simulink model "gm_opv_pluto_transmitter_HDL_coder_input"  (R2023a)
settings: Solver=FixedStepDiscrete  StartTime=0.0  StopTime=.02*40e-3  RelTol=1e-3
undefined symbols (not defined in the file or in its folder): bit_rate, bits_per_symbol, device_clock, PTTlength, symbol_rate
libraries: dsphdlsigops2 x2, hdlsllib x2, dspindex x1, commrandsrc3 x1
settings Model: Creator=matt  LastModifiedBy=matt
settings OptimizationCC: BlockReduction=off  ConditionallyExecuteInputs=off  DefaultParameterBehavior=Inlined
settings DebuggingCC: AlgebraicLoopMsg=error  InheritedTsInSrcMsg=none
settings HardwareCC: ProdBitPerPointer=32  ProdBitPerSizeT=32  ProdBitPerPtrDiffT=32  ProdLargestAtomicFloat=None  ProdIntDivRoundTo=Undefined  ProdEndianess=Unspecified  ProdWordSize=32  ProdHWDeviceType=ASIC/FPGA->ASIC/FPGA  TargetBitPerLong=64  TargetBitPerPointer=64  TargetBitPerSizeT=64  TargetBitPerPtrDiffT=64  TargetLongLongMode=on  TargetIntDivRoundTo=Zero  TargetEndianess=LittleEndian  TargetWordSize=64  TargetHWDeviceType=Custom Processor->MATLAB Host Computer  ProdEqTarget=off

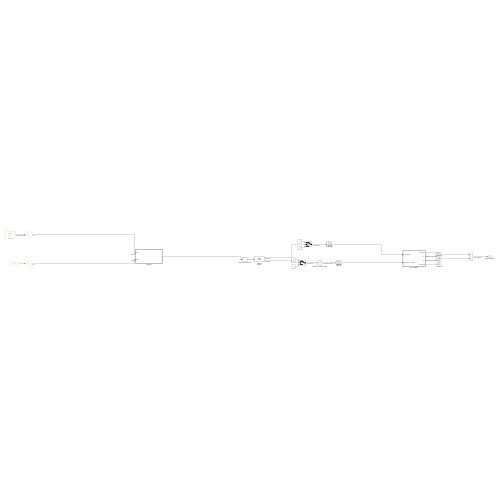
[thumbnail: Simulink's stored preview of the top-level diagram]
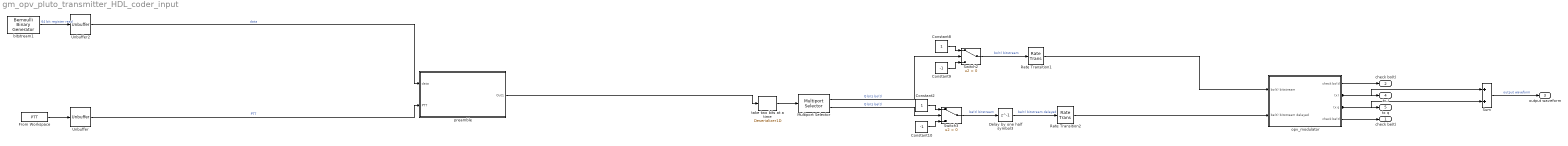
== system gm_opv_pluto_transmitter_HDL_coder_input ==
  Constant10 : Constant  Value=-1  OutDataTypeStr=fixdt(1,16,15)
  Constant2 : Constant  OutDataTypeStr=fixdt(1,16,15)
  Constant8 : Constant  OutDataTypeStr=fixdt(1,16,15)
  Constant9 : Constant  Value=-1  OutDataTypeStr=fixdt(1,16,15)
  Delay by one half symbol3 : Delay  DelayLength=1  SampleTime=1/(bits_per_symbol*symbol_rate)
  From Workspace : FromWorkspace  VariableName=PTT  SampleTime=PTTlength/(bit_rate)
  Multiport Selector : dspindex/Multiport Selector  rowsOrCols=Rows  idxCellArray={ 1, 2 }  idxErrMode=Clip Index
      settings: LibrarySourceBlock=|
      | dsphdlsupportsigmgmt/Multiport
      | Selector
  Rate Transition1 : RateTransition  Deterministic=off  OutPortSampleTime=1/device_clock
  Rate Transition2 : RateTransition  Deterministic=off  OutPortSampleTime=1/device_clock
  Sum : Sum  OutDataTypeStr=fixdt(1,16,15)  SaturateOnIntegerOverflow=on
  Switch2 : Switch  Criteria=u2 > Threshold  OutDataTypeStr=fixdt(1,16,15)  SaturateOnIntegerOverflow=off  InputSameDT=off
  Switch3 : Switch  Criteria=u2 > Threshold  OutDataTypeStr=fixdt(1,16,15)  SaturateOnIntegerOverflow=off  InputSameDT=off
  Unbuffer : Unbuffer
  Unbuffer2 : Unbuffer
  bitstream1 : commrandsrc3/Bernoulli Binary Generator  ProbabilityOfZero=0.5  SeedSource=Auto  Seed=0  SampleTime=(1/bit_rate)  SamplesPerFrame=64  OutputDataType=boolean  SimulateUsing=Interpreted execution
  opv_modulator : Subsystem  TreatAsAtomicUnit=on
  preamble : Subsystem  TreatAsAtomicUnit=on
  take two bits at a time : hdlsllib/HDL Operations/Deserializer1D  Ratio=2  IdleCycles=0  InitialCondition=0  startIn=off  validIn=off  validOut=off  inputDataDimensions=-1  inputSampleTime=-1  inputSignalType=auto
  check be(t) : Outport
  "check bo(t) " : Outport  Port=2
  output waveform : Outport  Port=3
  tx I : Outport  Port=4
  tx q : Outport  Port=5
  wires:
  preamble/1(Out1) -> take two bits at a time/1
  Unbuffer/1 -> preamble/2(PTT)  "PTT"
  Unbuffer2/1 -> preamble/1(data)  "data"
  opv_modulator/4(check be(t)) -> check be(t)/1
  opv_modulator/3(tx q) -> tx q/1, Sum/2
  opv_modulator/2(tx I) -> tx I/1, Sum/1
  opv_modulator/1("check bo(t) ") -> "check bo(t) "/1
  Rate Transition2/1 -> opv_modulator/2(be(t) bitstream delayed)
  Rate Transition1/1 -> opv_modulator/1(bo(t) bitstream)
  bitstream1/1 -> Unbuffer2/1  "64 bit register read"
  Constant2/1 -> Switch3/1
  Constant10/1 -> Switch3/3
  Constant9/1 -> Switch2/3
  Constant8/1 -> Switch2/1
  Multiport Selector/2 -> Switch3/2  "Q bits be(t)"
  Multiport Selector/1 -> Switch2/2  "Q bits bo(t)"
  take two bits at a time/1 -> Multiport Selector/1
  From Workspace/1 -> Unbuffer/1
  Delay by one half symbol3/1 -> Rate Transition2/1  "be(t) bitstream delayed"
  Sum/1 -> output waveform/1  "output waveform"
  Switch3/1 -> Delay by one half symbol3/1  "be(t) bitstream"
  Switch2/1 -> Rate Transition1/1  "bo(t) bitstream"

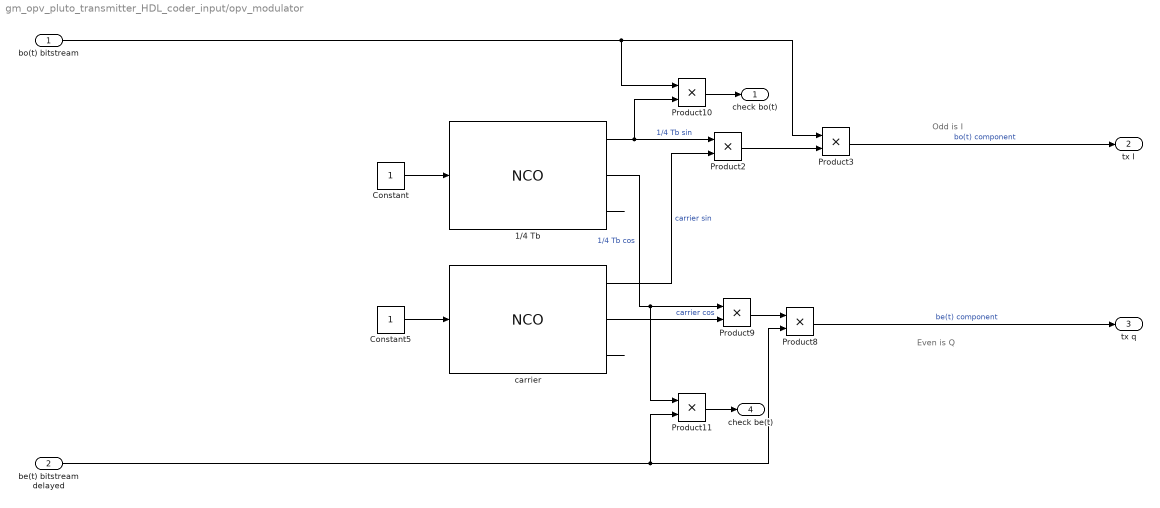
== system gm_opv_pluto_transmitter_HDL_coder_input/opv_modulator ==
  note: Odd is I
  note: Even is Q
  bo(t) bitstream : Inport
  be(t) bitstream delayed : Inport  Port=2
  1/4 Tb : dsphdlsigops2/NCO  PhaseIncrementSource=Property  PhaseIncrement=phase_increment_bo_be  PhaseOffsetSource=Property  PhaseOffset=phase_offset  DitherSource=None  NumDitherBits=dither_bits  SamplesPerFrame=1  LUTCompress=on  ResetAction=off  Waveform=Sine and cosine  PhasePort=off  SimulateUsing=Code generation  AccumulatorWL=accumulator_width  PhaseQuantization=on  NumQuantizerAccumulatorBits=quantizer_word_length  OutputDataType=Binary point scaling  OutputWL=16  OutputFL=15
      settings: LibrarySourceBlock=dsphdlsrcs2/NCO
  Constant : Constant  OutDataTypeStr=boolean
  Constant5 : Constant  OutDataTypeStr=boolean
  Product{2..3,8..11} (6 alike) : Product  OutDataTypeStr=fixdt(1,16,15)
  carrier : dsphdlsigops2/NCO  PhaseIncrementSource=Property  PhaseIncrement=phase_increment_carrier  PhaseOffsetSource=Property  PhaseOffset=phase_offset  DitherSource=None  NumDitherBits=dither_bits  SamplesPerFrame=1  LUTCompress=on  ResetAction=off  Waveform=Sine and cosine  PhasePort=off  SimulateUsing=Code generation  AccumulatorWL=accumulator_width  PhaseQuantization=on  NumQuantizerAccumulatorBits=quantizer_word_length  OutputDataType=Binary point scaling  OutputWL=16  OutputFL=15
      settings: LibrarySourceBlock=dsphdlsrcs2/NCO
  "check bo(t) " : Outport
  tx I : Outport  Port=2
  tx q : Outport  Port=3
  check be(t) : Outport  Port=4
  wires:
  Product2/1 -> Product3/2
  Product9/1 -> Product8/1
  carrier/2 -> Product9/2  "carrier cos"
  carrier/1 -> Product2/2  "carrier sin"
  1/4 Tb/2 -> Product9/1, Product11/1  "1/4 Tb cos"
  1/4 Tb/1 -> Product2/1, Product10/2  "1/4 Tb sin"
  Product3/1 -> tx I/1  "bo(t) component"
  Product8/1 -> tx q/1  "be(t) component"
  Constant5/1 -> carrier/1
  Constant/1 -> 1/4 Tb/1
  be(t) bitstream delayed/1 -> Product8/2, Product11/2
  carrier/3 -> ?
  1/4 Tb/3 -> ?
  bo(t) bitstream/1 -> Product3/1, Product10/1
  Product10/1 -> "check bo(t) "/1
  Product11/1 -> check be(t)/1

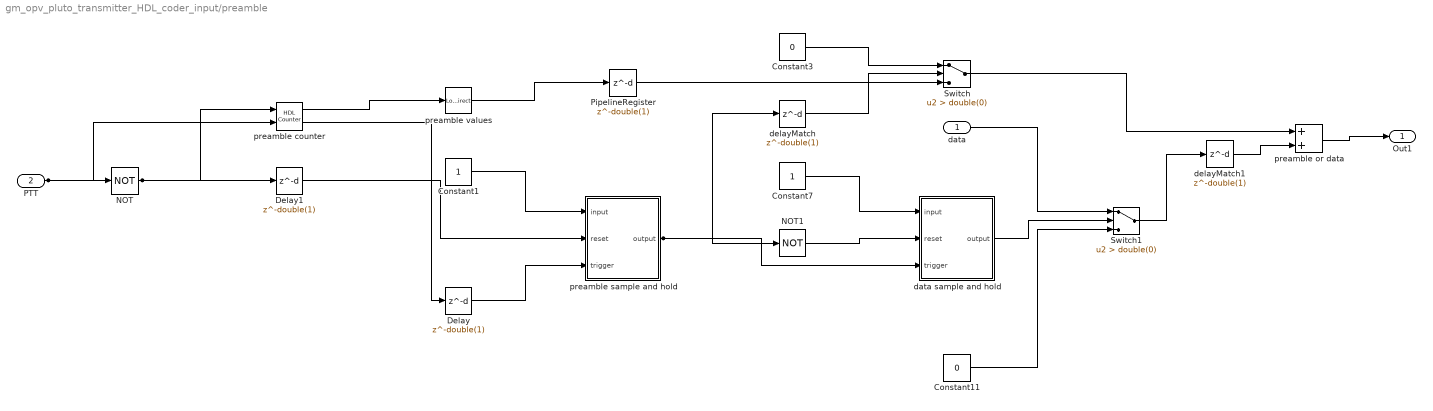
== system gm_opv_pluto_transmitter_HDL_coder_input/preamble ==
  data : Inport  OutDataTypeStr=boolean  PortDimensions=1  SampleTime=1.8450184501845e-05
  PTT : Inport  Port=2  OutDataTypeStr=boolean  PortDimensions=1  SampleTime=1.8450184501845e-05
  Constant1 : Constant  OutDataTypeStr=boolean  SampleTime=1.8450184501845e-05
  Constant11 : Constant  Value=0  VectorParams1D=off  OutDataTypeStr=boolean  SampleTime=1.8450184501845e-05
  Constant3 : Constant  Value=0  VectorParams1D=off  OutDataTypeStr=boolean  SampleTime=1.8450184501845e-05
  Constant7 : Constant  OutDataTypeStr=boolean  SampleTime=1.8450184501845e-05
  Delay : Delay  DelayLength=double(1)  InitialCondition=0  SampleTime=1.8450184501845e-05
  Delay1 : Delay  DelayLength=double(1)  InitialCondition=0  SampleTime=1.8450184501845e-05
  NOT : Logic  Operator=NOT  Inputs=1  AllPortsSameDT=off  OutDataTypeStr=boolean  SampleTime=1.8450184501845e-05
  NOT1 : Logic  Operator=NOT  Inputs=1  AllPortsSameDT=off  OutDataTypeStr=boolean  SampleTime=1.8450184501845e-05
  PipelineRegister : Delay  DelayLength=double(1)  InitialCondition=0  SampleTime=1.8450184501845e-05
  Switch : Switch  Criteria=u2 > Threshold  Threshold=double(0)  OutDataTypeStr=boolean  SampleTime=1.8450184501845e-05  SaturateOnIntegerOverflow=off  InputSameDT=off
  Switch1 : Switch  Criteria=u2 > Threshold  Threshold=double(0)  OutDataTypeStr=boolean  SampleTime=1.8450184501845e-05  SaturateOnIntegerOverflow=off  InputSameDT=off
  data sample and hold : Subsystem
  delayMatch : Delay  DelayLength=double(1)  InitialCondition=0  SampleTime=1.8450184501845e-05
  delayMatch1 : Delay  DelayLength=double(1)  InitialCondition=0  SampleTime=1.8450184501845e-05
  preamble counter : hdlsllib/Sources/HDL Counter  CountType=Count limited  CountInit=0  CountStep=1  CountMax=2168  CountFromType=Initial value  CountFrom=0  CountResetPort=on  CountLoadPort=off  CountEnbPort=on  CountDirPort=off  CountHitOutputPort=on  CountDataType=Unsigned  CountWordLen=16  CountFracLen=0  CountSampTime=1
  preamble or data : Sum  AccumDataTypeStr=fixdt(0, 9, 0)  OutDataTypeStr=fixdt(0, 9, 0)  SampleTime=1.8450184501845e-05
  preamble sample and hold : Subsystem
  preamble values : LookupNDDirect  NumberOfTableDimensions=1  Table="reshape(logical([0 1 1 0 0 1 1 0 0 1 1 0 0 1 1 0 0 1 1 0 0 1 1 0 0 1 1 0 0 1 1 0 0 1 1 0 0 1 1 0 0 1 1 0 0 1 1 0 0 1 1 0 0 1 1 0 0 1 1 0 0 1 1 0 0 1 1 0 0 1 1 0 0 1 1 0 0 1 1 0 0 1 1 0 0 1 1 0 0 1 1 0 0 1 1 0 0 1 1 0 0 1 1 0 0 1 1 0 0 1 1 0 0 1 1 0 0 1 1 0 0 1 1 0 0 1 1 0 0 1 1 0 0 1 1 0 0 1 1 0 0 1 1 0 0 1 1 0 0 1 1 0 0 1 1 0 0 1 1 0 0 1 1 0 0 1 1 0 0 1 1 0 0 1 1 0 0 1 1 0 0 1 1 0 0 1 1 0 0 1 1 0 0 1 1 0 0 1 1 0 0 1 1 0 0 1 1 0 0 1 1 0 0 1 1 0 0 1 1 0 0 1 1 0 0 1 1 0 0 1 1 0 0 1 1 0 0 1 1 0 0 1 1 0 0 1 1 0 0 1 1 0 0 1 1 0 0 1 1 0 0 1 1 0 0 1 1 0 0 1 1 0 0 1 1 0 0 1 1 0 0 1 1 0 0 1 1 0 0 1 1 0 0 1 1 0 0 1 1 0 0 1 1 0 0 1 1 0 0 1 1 0 0 1 1 0 0 1 1 0 0 1 1 0 0 1 1 0 0 1 1 0 0 1 1 0 0 1 1 0 0 1 1 0 0 1 1 0 0 1 1 0 0 1 1 0 0 1 1 0 0 1 1 0 0 1 1 0 0 1 1 0 0 1 1 0 0 1 1 0 0 1 1 0 0 1 1 0 0 1 1 0 0 1 1 0 0 1 1 0 0 1 1 0 0 1 1 0 0 1 1 0 0 1 1 0 0 1 1 0 0 1 1 0 0 1 1 0 0 1 1 0 0 1 1 0 0 1 1 0 0 1 1 0 0 1 1 0 0 1 1 0 0 1 1 0 0 1 1 0 0 1 1 0 0 1 1 0 0 1 1 0 0 1 1 0 0 1 1 0 0 1 1 0 0 1 1 0 0 1 1 0 0 1 1 0 0 1 1 0 0 1 1 0 0 1 1 0 0 1 1 0 0 1 1 0 0 1 1 0 0 1 1 0 0 1 1 0 0 1 1 0 0 1 1 0 0 1 1 0 0 1 1 0 0 1 1 0 0 1 1 0 0 1 1 0 0 1 1 0 0 1 1 0 0 1 1 0 0 1 1 0 0 1 1 0 0 1 1 0 0 1 1 0 0 1 1 0 0 1 1 0 0 1 1 0 0 1 1 0 0 1 1 0 0 1 1 0 0 1 1 0 0 1 1 0 0 1 1 0 0 1 1 0 0 1 1 0 0 1 1 0 0 1 1 0 0 1 1 0 0 1 1 0 0 1 1 0 0 1 1 0 0 1 1 0 0 1 1 0 0 1 1 0 0 1 1 0 0 1 1 0 0 1 1 0 0 1 1 0 0 1 1 0 0 1 1 0 0 1 1 0 0 1 1 0 0 1 1 0 0 1 1 0 0 1 1 0 0 1 1 0 0 1 1 0 0 1 1 0 0 1 1 0 0 1 1 0 0 1 1 0 0 1 1 0 0 1 1 0 0 1 1 0 0 1 1 0 0 1 1 0 0 1 1 0 0 1 1 0 0 1 1 0 0 1 1 0 0 1 1 0 0 1 1 0 0 1 1 0 0 1 1 0 0 1 1 0 0 1 1 0 0 1 1 0 0 1 1 0 0 1 1 0 0 1 1 0 0 1 1 0 0 1 1 0 0 1 1 0 0 1 1 0 0 1 1 0 0 1 1 0 0 1 1 0 0 1 1 0 0 1 1 0 0 1 1 0 0 1 1 0 0 1 1 0 0 1 1 0 0 1 1 0 0 1 1 0 0 1 1 0 0 1 1 0 0 1 1 0 0 1 1 0 0 1 1 0 0 1 1 0 0 1 1 0 0 1 1 0 0 1 1 0 0 1 1 0 0 1 1 0 0 1 1 0 0 1 1 0 0 1 1 0 0 1 1 0 0 1 1 0 0 1 1 0 0 1 1 0 0 1 1 0 0 1 1 0 0 1 1 0 0 1 1 0 0 1 1 0 0 1 1 0 0 1 1 0 0 1 1 0 0 1 1 0 0 1 1 0 0 1 1 0 0 1 1 0 0 1 1 0 0 1 1 0 0 1 1 0 0 1 1 0 0 1 1 0 0 1 1 0 0 1 1 0 0 1 1 0 0 1 1 0 0 1 1 0 0 1 1 0 0 1 1 0 0 1 1 0 0 1 1 0 0 1 1 0 0 1 1 0 0 1 1 0 0 1 1 0 0 1 1 0 0 1 1 0 0 1 1 0 0 1 1 0 0 1 1 0 0 1 1 0 0 1 1 0 0 1 1 0 0 1 1 0 0 1 1 0 0 1 1 0 0 1 1 0 0 1 1 0 0 1 1 0 0 1 1 0 0 1 1 0 0 1 1 0 0 1 1 0 0 1 1 0 0 1 1 0 0 1 1 0 0 1 1 0 0 1 1 0 0 1 1 0 0 1 1 0 0 1 1 0 0 1 1 0 0 1 1 0 0 1 1 0 0 1 1 0 0 1 1 0 0 1 1 0 0 1 1 0 0 1 1 0 0 1 1 0 0 1 1 0 0 1 1 0 0 1 1 0 0 1 1 0 0 1 1 0 0 1 1 0 0 1 1 0 0 1 1 0 0 1 1 0 0 1 1 0 0 1 1 0 0 1 1 0 0 1 1 0 0 1 1 0 0 1 1 0 0 1 1 0 0 1 1 0 0 1 1 0 0 1 1 0 0 1 1 0 0 1 1 0 0 1 1 0 0 1 1 0 0 1 1 0 0 1 1 0 0 1 1 0 0 1 1 0 0 1 1 0 0 1 1 0 0 1 1 0 0 1 1 0 0 1 1 0 0 1 1 0 0 1 1 0 0 1 1 0 0 1 1 0 0 1 1 0 0 1 1 0 0 1 1 0 0 1 1 0 0 1 1 0 0 1 1 0 0 1 1 0 0 1 1 0 0 1 1 0 0 1 1 0 0 1 1 0 0 1 1 0 0 1 1 0 0 1 1 0 0 1 1 0 0 1 1 0 0 1 1 0 0 1 1 0 0 1 1 0 0 1 1 0 0 1 1 0 0 1 1 0 0 1 1 0 0 1 1 0 0 1 1 0 0 1 1 0 0 1 1 0 0 1 1 0 0 1 1 0 0 1 1 0 0 1 1 0 0 1 1 0 0 1 1 0 0 1 1 0 0 1 1 0 0 1 1 0 0 1 1 0 0 1 1 0 0 1 1 0 0 1 1 0 0 1 1 0 0 1 1 0 0 1 1 0 0 1 1 0 0 1 1 0 0 1 1 0 0 1 1 0 0 1 1 0 0 1 1 0 0 1 1 0 0 1 1 0 0 1 1 0 0 1 1 0 0 1 1 0 0 1 1 0 0 1 1 0 0 1 1 0 0 1 1 0 0 1 1 0 0 1 1 0 0 1 1 0 0 1 1 0 0 1 1 0 0 1 1 0 0 1 1 0 0 1 1 0 0 1 1 0 0 1 1 0 0 1 1 0 0 1 1 0 0 1 1 0 0 1 1 0 0 1 1 0 0 1 1 0 0 1 1 0 0 1 1 0 0 1 1 0 0 1 1 0 0 1 1 0 0 1 1 0 0 1 1 0 0 1 1 0 0 1 1 0 0 1 1 0 0 1 1 0 0 1 1 0 0 1 1 0 0 1 1 0 0 1 1 0 0 1 1 0 0 1 1 0 0 1 1 0 0 1 1 0 0 1 1 0 0 1 1 0 0 1 1 0 0 1 1 0 0 1 1 0 0 1 1 0 0 1 1 0 0 1 1 0 0 1 1 0 0 1 1 0 0 1 1 0 0 1 1 0 0 1 1 0 0 1 1 0 0 1 1 0 0 1 1 0 0 1 1 0 0 1 1 0 0 1 1 0 0 1 1 0 0 1 1 0 0 1 1 0 0 1 1 0 0 1 1 0 0 1 1 0 0 1 1 0 0 1 1 0 0 1 1 0 0 1 1 0 0 1 1 0 0 1 1 0 0 1 1 0 0 1 1 0 0 1 1 0 0 1 1 0 0 1 1 0 0 1 1 0 0 1 1 0 0 1 1 0 0 1 1 0 0 1 1 0 0 1 1 0 0 1 1 0 0 1 1 0 0 1 1 0 0 1 1 0 0 1 1 0 0 1 1 0 0 1 1 0 0 1 1 0 0 1 1 0 0 1 1 0 0 1 1 0 0 1 1 0 0 1 1 0 0 1 1 0 0 1 1 0 0 1 1 0 0 1 1 0 0 1 1 0 0 1 1 0 0 1 1 0 0 1 1 0 0 1 1 0 0 1 1 0 0 1 1 0 0 1 1 0 0 1 1 0 0 1 1 0 0 1 1 0 0 1 1 0 0 1 1 0 0 1 1 0 0 1 1 0 0 1 1 0 0 1 1 0 0 1 1 0 0 1 1 0 0 1 1 0 0 1 1 0 0 1 1 0 0 1 1 0 0 1 1 0 0 1 1 0 0 1 1 0 0 1 1 0 0 1 1 0 0 1 1 0 0 1 1 0 0 1 1 0 0 1 1 0 0 1 1 0 0 1 1 0 0 1 1 0 0 1 1 0 0 1 1 0 0 1 1 0 0 1 1 0 0 1 1 0 0 1 1 0 0 1 1 0 0 1 1 0 0 1 1 0 0 1 1 0 0 1 1 0 0 1 1 0 0 1 1 0 0 1 1 0 0 1 1 0 0 1 1 0 0 1 1 0 0 1 1 0 0 1 1 0 0]).', [2169     1])"  DiagnosticForOutOfRangeInput=Error  SampleTime=1.8450184501845e-05  TableDataTypeStr=boolean
  Out1 : Outport  SampleTime=1.8450184501845e-05
  wires:
  data/1 -> Switch1/1
  PTT/1 -> NOT/1, preamble counter/2
  Constant1/1 -> preamble sample and hold/1(input)
  Constant11/1 -> Switch1/3
  Constant3/1 -> Switch/1
  Constant7/1 -> data sample and hold/1(input)
  Delay/1 -> preamble sample and hold/3(trigger)
  Delay1/1 -> preamble sample and hold/2(reset)
  NOT/1 -> Delay1/1, preamble counter/1
  NOT1/1 -> data sample and hold/2(reset)
  Switch/1 -> preamble or data/1
  delayMatch1/1 -> preamble or data/2
  data sample and hold/1(output) -> Switch1/2
  preamble counter/1 -> preamble values/1
  preamble counter/2 -> Delay/1
  preamble or data/1 -> Out1/1
  delayMatch/1 -> Switch/2
  PipelineRegister/1 -> Switch/3
  preamble sample and hold/1(output) -> delayMatch/1, NOT1/1, data sample and hold/3(trigger)
  Switch1/1 -> delayMatch1/1
  preamble values/1 -> PipelineRegister/1

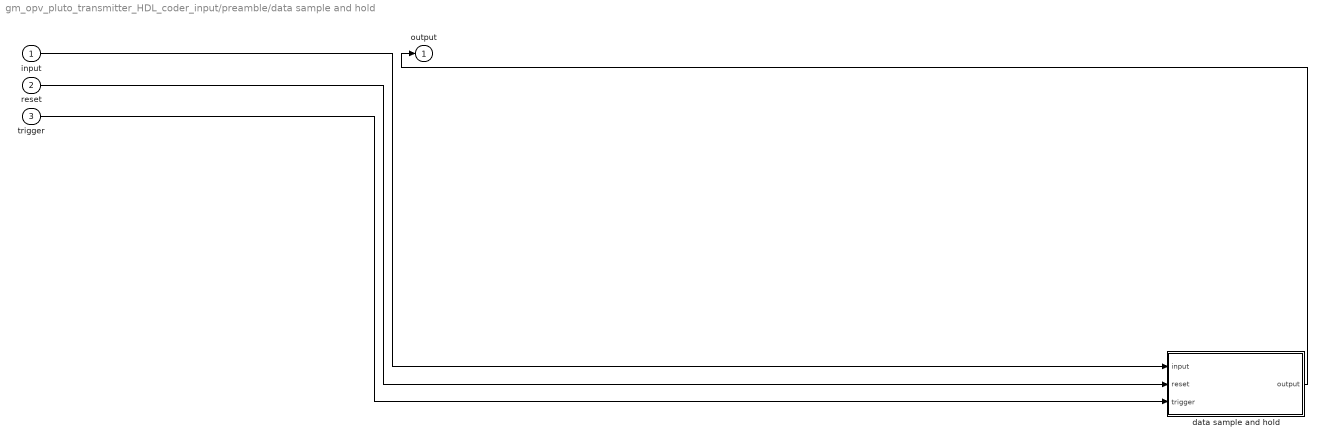
== system gm_opv_pluto_transmitter_HDL_coder_input/preamble/data sample and hold ==
  input : Inport  OutDataTypeStr=boolean  PortDimensions=1  SampleTime=1.8450184501845e-05
  reset : Inport  Port=2  OutDataTypeStr=boolean  PortDimensions=1  SampleTime=1.8450184501845e-05
  trigger : Inport  Port=3  OutDataTypeStr=boolean  PortDimensions=1  SampleTime=1.8450184501845e-05
  data sample and hold : MATLAB Function  TreatAsAtomicUnit=on
  output : Outport  SampleTime=1.8450184501845e-05  VectorParamsAs1DForOutWhenUnconnected=off
  wires:
  data sample and hold/1(output) -> output/1
  input/1 -> data sample and hold/1(input)
  reset/1 -> data sample and hold/2(reset)
  trigger/1 -> data sample and hold/3(trigger)

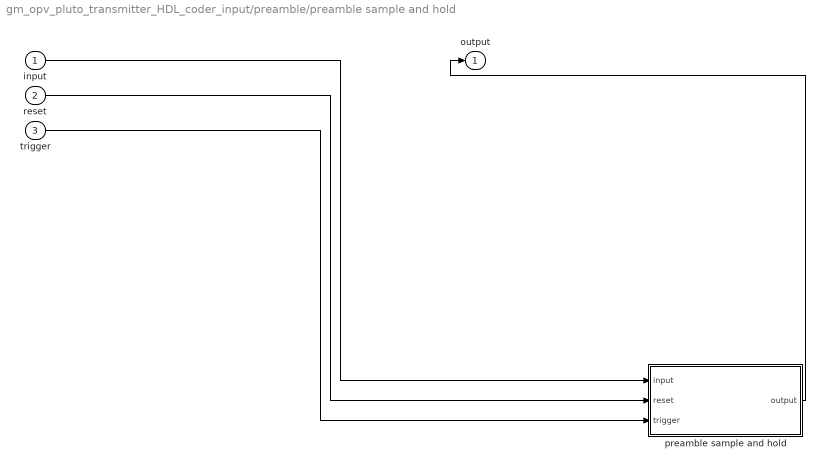
== system gm_opv_pluto_transmitter_HDL_coder_input/preamble/preamble sample and hold ==
  input : Inport  OutDataTypeStr=boolean  PortDimensions=1  SampleTime=1.8450184501845e-05
  reset : Inport  Port=2  OutDataTypeStr=boolean  PortDimensions=1  SampleTime=1.8450184501845e-05
  trigger : Inport  Port=3  OutDataTypeStr=boolean  PortDimensions=1  SampleTime=1.8450184501845e-05
  preamble sample and hold : MATLAB Function  TreatAsAtomicUnit=on
  output : Outport  SampleTime=1.8450184501845e-05  VectorParamsAs1DForOutWhenUnconnected=off
  wires:
  preamble sample and hold/1(output) -> output/1
  input/1 -> preamble sample and hold/1(input)
  reset/1 -> preamble sample and hold/2(reset)
  trigger/1 -> preamble sample and hold/3(trigger)

== matlab function gm_opv_pluto_transmitter_HDL_coder_input/preamble/data sample and hold/data sample and hold ==
  data: input input; output output; reset input; trigger input
function output   = resettable_sample_and_hold(input, reset, trigger)
%#codegen

%Resettable Sample and Hold Circuit
% This was written because S&H within Resettable Subsystems in Simulink
% is not supported by HDL Coder. We needed this functionality, so this
% custom function was written. 



initial_value = false;

    persistent sample_held;
    if isempty(sample_held)
        sample_held = false;
    end

    persistent output_held_value;
    if isempty(output_held_value)
        output_held_value = false;
    end


switch reset
    case 0 % not in reset
        switch trigger
            case 0
                output = output_held_value;
            case 1
                if sample_held == false
                    output_held_value = input;
                    output = output_held_value;
                    sample_held = true;
                else
                    output = output_held_value;
                end
            otherwise
                output = initial_value;
        end
    case 1 % reset signal received
        output = initial_value;
        sample_held = false;
        output_held_value = false;
    otherwise
        output = initial_value;
        
end

== matlab function gm_opv_pluto_transmitter_HDL_coder_input/preamble/preamble sample and hold/preamble sample and hold ==
  data: input input; output output; reset input; trigger input
function output   = resettable_sample_and_hold(input, reset, trigger)
%#codegen

%Resettable Sample and Hold Circuit
% This was written because S&H within Resettable Subsystems in Simulink
% is not supported by HDL Coder. We needed this functionality, so this
% custom function was written. 



initial_value = false;

    persistent sample_held;
    if isempty(sample_held)
        sample_held = false;
    end

    persistent output_held_value;
    if isempty(output_held_value)
        output_held_value = false;
    end


switch reset
    case 0 % not in reset
        switch trigger
            case 0
                output = output_held_value;
            case 1
                if sample_held == false
                    output_held_value = input;
                    output = output_held_value;
                    sample_held = true;
                else
                    output = output_held_value;
                end
            otherwise
                output = initial_value;
        end
    case 1 % reset signal received
        output = initial_value;
        sample_held = false;
        output_held_value = false;
    otherwise
        output = initial_value;
        
end
